simulink model "uz_mpc_3ph"  (R2021a)
settings: Solver=FixedStepDiscrete  StartTime=0.0  StopTime=2000*t_ADC  RelTol=1e-3
values from neighbouring files (symbols this model uses):
  IB = sqrt(2)*IR    [uz_mpc_3ph_init.m]
  id_ref = 0.0    (= 0)    [uz_mpc_3ph_init.m]
  iq_ref = 2.0    (= 2)    [uz_mpc_3ph_init.m]
  lambda_d = 1.0    (= 1)    [uz_mpc_3ph_init.m]
  lambda_q = 1.0    (= 1)    [uz_mpc_3ph_init.m]
  lambda_u = 0.000013    (= 1.3e-05)    [uz_mpc_3ph_init.m]
  Ld_over_LB = Ld/LB    [uz_mpc_3ph_init.m]
  Lq_over_LB = Lq/LB    [uz_mpc_3ph_init.m]
  n_rpm = 250.0    (= 250)    [uz_mpc_3ph_init.m]
  omegaB = nR*2*pi()/60*p    [uz_mpc_3ph_init.m]
  p = 4    [uz_mpc_3ph_init.m]
  psi_pm_over_psiB = psi_pm/psiB    [uz_mpc_3ph_init.m]
  Rs_over_ZB = Rs/ZB    [uz_mpc_3ph_init.m]
  t_ADC = 1/f_ADC    (= 1e-05)    [uz_mpc_3ph_init.m]
  t_clock = 1/f_clock    (= 1e-08)    [uz_mpc_3ph_init.m]
  Ts_times_ZB_over_Ld = Ts*ZB/Ld    [uz_mpc_3ph_init.m]
  Ts_times_ZB_over_Lq = Ts*ZB/Lq    [uz_mpc_3ph_init.m]
  v_dc = 48.0    (= 48)    [uz_mpc_3ph_init.m]
  VB = sqrt(2/3)*VR    [uz_mpc_3ph_init.m]
libraries: nesl_utility x19, simulink x18, fl_lib x15, ee_lib x7, hdlsllib x2, spsAlphaBetaZerotodq0Lib x1
(part 2 of 3)

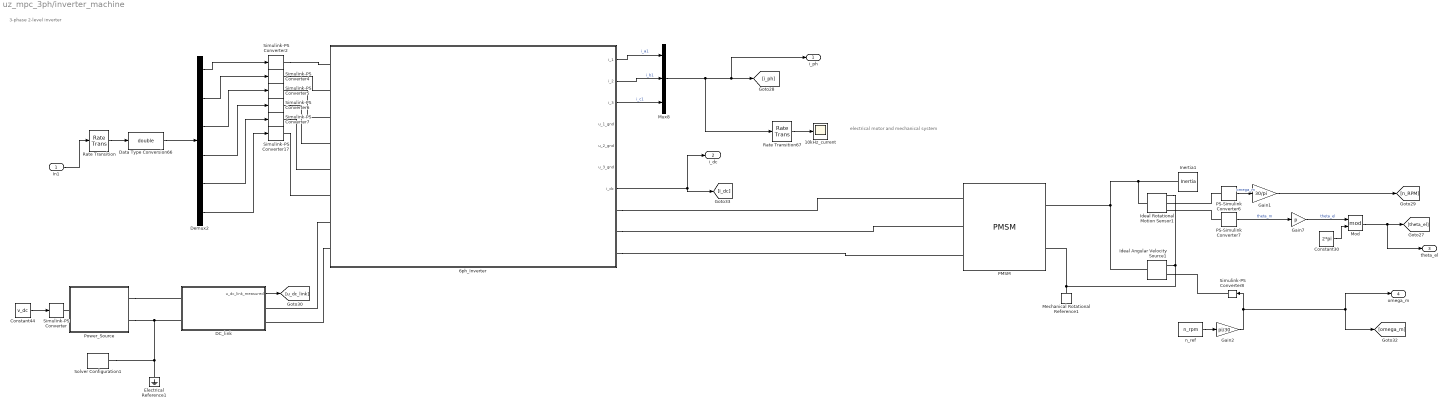
== system uz_mpc_3ph/inverter_machine ==
  note: electrical motor and mechanical system
  note: 3-phase 2-level inverter
  In1 : Inport
  10kHz_current : Scope
  6ph_Inverter : Subsystem
  Constant30 : Constant  Value=2*pi  SampleTime=-1
  Constant44 : Constant  Value=v_dc  SampleTime=-1
  DC_link : Subsystem
  Data Type Conversion66 : DataTypeConversion  OutDataTypeStr=double
  Demux2 : Demux  Outputs=6
  Electrical Reference1 : fl_lib/Electrical/Electrical Elements/Electrical Reference
  Gain1 : Gain  Gain=30/pi
  Gain2 : Gain  Gain=pi/30
  Gain7 : Gain  Gain=p
  Ideal Angular Velocity Source1 : fl_lib/Mechanical/Mechanical Sources/Ideal Angular Velocity Source
  Ideal Rotational Motion Sensor1 : fl_lib/Mechanical/Mechanical Sensors/Ideal Rotational Motion Sensor  wrap_angle=simscape.enum.onoff.off  offset=0 deg
  Inertia1 : fl_lib/Mechanical/Rotational Elements/Inertia  inertia=J kg*m^2  num_ports=foundation.enum.numPorts2.one  w_specify=off  w_priority=High  w=0 rad/s  w_nominal_specify=off  w_nominal_unit=rad/s  w_nominal_value=1  t_specify=off  t_priority=None  t=0 N*m  t_nominal_specify=off  t_nominal_unit=N*m  t_nominal_value=1
  Mechanical Rotational Reference1 : fl_lib/Mechanical/Rotational Elements/Mechanical Rotational Reference
  Mod : Math  Operator=mod  SaturateOnIntegerOverflow=on
  Mux8 : Mux  Inputs=3
  PMSM : ee_lib/Electromechanical/Permanent Magnet/PMSM  winding_type=ee.enum.statorconnection.wye  machine_param=ee.enum.pmsm.parameterization.constant  nPolePairs=p  pmflux_param=ee.enum.pmflux.fluxlinkage  pm_flux_linkage=psi_pm Wb  torque_constant=0.18 N*m/A  back_emf_constant=0.18 V/(rad/s)  stator_param=ee.enum.statorparam.LdLqL0  Ld=Ld H  Lq=Lq H  idVec=[-200, 0, 200] A  iqVec=[-200, 0, 200] A  LdMatrix=0.0002 * ones(3, 3) H  LqMatrix=0.0002 * ones(3, 3) H  PmMatrix=0.1 * ones(3, 3) Wb  ktMatrix=0.18 * ones(3, 3) N*m/A  keMatrix=0.18 * ones(3, 3) V/(rad/s)  L0=0.00016 H  Ls=0.0002 H  Lm=-0.00002 H  Ms=0.00002 H  Rs=Rs Ohm  zero_sequence=ee.enum.park.zerosequence.exclude  J=0.01 kg*m^2  lam=0 N*m/(rad/s)  axes_param=ee.enum.rotorangle.daxis  i_d_specify=off  i_d_priority=None  i_d=0 A  i_d_nominal_specify=off  i_d_nominal_unit=A  i_d_nominal_value=1  i_q_specify=off  i_q_priority=None  i_q=0 A  i_q_nominal_specify=off  i_q_nominal_unit=A  i_q_nominal_value=1  torque_specify=off  torque_priority=None  torque=0 N*m  torque_nominal_specify=off  torque_nominal_unit=N*m  torque_nominal_value=1  angular_velocity_specify=off  angular_velocity_priority=High  angular_velocity=0 rpm  angular_velocity_nominal_specify=off  angular_velocity_nominal_unit=rpm  angular_velocity_nominal_value=1  angular_position_specify=off  angular_position_priority=High  angular_position=0 deg  angular_position_nominal_specify=off  angular_position_nominal_unit=deg  angular_position_nominal_value=1  loss_param=ee.enum.ironloss.none  losses_oc=[0, 0, 0] W  losses_sc=[0, 0, 0] W  f_losses=60 Hz  Isc_losses=95 A  Tmeas=298.15 K  alpha=3.93e-3 1/K  alpha_flux=-0.001 1/K  stator_thermal_mass=100 J/K  rotor_thermal_mass=200 J/K  Rm_percent_rotor=90  Rd_percent_rotor=30  temperatureA_specify=off  temperatureA_priority=High  temperatureA=25 degC  temperatureA_nominal_specify=off  temperatureA_nominal_unit=degC  temperatureA_nominal_value=1  temperatureB_specify=off  temperatureB_priority=High  temperatureB=25 degC  temperatureB_nominal_specify=off  temperatureB_nominal_unit=degC  temperatureB_nominal_value=1  temperatureC_specify=off  temperatureC_priority=High  temperatureC=25 degC  temperatureC_nominal_specify=off  temperatureC_nominal_unit=degC  temperatureC_nominal_value=1  temperatureR_specify=off  temperatureR_priority=High  temperatureR=25 degC  temperatureR_nominal_specify=off  temperatureR_nominal_unit=degC  temperatureR_nominal_value=1
      settings: InternalSimscapePortConfiguration="{\"Bottom\":[],\"Left\":[{\"id\":\"a\",\"label\":\"a\",\"type\":\"foundation.electrical.electrical\"},{\"id\":\"b\",\"label\":\"b\",\"type\":\"foundation.electrical.electrical\"},{\"id\":\"c\",\"label\":\"c\",\"type\":\"foundation.electrical.electrical\"}],\"Right\":[{\"id\":\"R\",\"label\":\"R\",\"type\":\"foundation.mechanical.rotational.rotational\"},{\"id\":\"C\",\"label\":\"C\",\"type\":\"foundation.mechanical.rotational.rotational\"}],\"Top\":[]}"
  PS-Simulink Converter6 : nesl_utility/PS-Simulink Converter  PhysicalDomain=network_engine_domain  SubClassName=ps_output  LeftPortType=input  RightPortType=output  PseudoPeriodic=off  Frequencies=[]  Unit=1  AffineConversion=off
      settings: SourceProductBaseCode=PW,SS
  PS-Simulink Converter7 : nesl_utility/PS-Simulink Converter  PhysicalDomain=network_engine_domain  SubClassName=ps_output  LeftPortType=input  RightPortType=output  PseudoPeriodic=off  Frequencies=[]  Unit=1  AffineConversion=off
      settings: SourceProductBaseCode=PW,SS
  Power_Source : Subsystem
  Rate Transition : RateTransition  OutPortSampleTime=1e-6
  Rate Transition67 : RateTransition  OutPortSampleTime=0.0001
  Simulink-PS Converter{,2,4..8,17} (8 alike) : nesl_utility/Simulink-PS Converter  PhysicalDomain=network_engine_domain  SubClassName=ps_input  LeftPortType=input  RightPortType=output  PseudoPeriodic=off  Frequencies=[]  NoiseDistribution=none  NoiseParameters=[]  Unit=1  AffineConversion=off  FilteringAndDerivatives=provide  SimscapeFilterOrder=1  InputFilterTimeConstant=0.001  UdotUserProvided=0
      Simulink-PS Converter settings: SourceProductBaseCode=PW,SS
      Simulink-PS Converter8 settings: SourceProductBaseCode=PW,SS
  Solver Configuration1 : nesl_utility/Solver Configuration  PhysicalDomain=network_engine_domain  SubClassName=solver  LeftPortType=input  RightPortType=generic  Tones=[]  Harmonics=[]  SimulateNoise=off  Profile=off  UseLocalSampling=off  EnableSwitchedLinearOptims=on  FrequencyDomain=off  UseCCode=off  RelTol=0.001  AbsTol=1e-06  MinStep=1e-09  ToWorkspace=off  RevertToSquareIcSolve=off  NumHomotopyIterations=100  PhasorMode=off  PhasorModeNumHarmonics=1  DoDC=off  ResidualTolerance=1e-09  UseLocalSolver=on  LocalSolverChoice=NE_BACKWARD_EULER_ADVANCER  LocalSolverSampleTime=1e-6  DoFixedCost=on  MaxNonlinIter=3  MaxModeIter=2  ComputeImpulses=off  ImpulseIterations=2  LinearAlgebra=Sparse  EquationFormulation=NE_TIME_EF  DelaysMemoryBudget=1024  AutomaticFiltering=on  FilteringTimeConstant=0.001  PartitionStorageMethod=AS_NEEDED  PartitionMemoryBudget=1024  PartitionMethod=FAST
      settings: SourceProductBaseCode=PW,SS
  n_ref : Constant  Value=n_rpm  SampleTime=-1
  i_ph : Outport
  i_dc : Outport  Port=2
  theta_el : Outport  Port=3
  omega_m : Outport  Port=4
  wires:
  Mux8/1 -> Rate Transition67/1, i_ph/1, [i_ph]
  Gain2/1 -> [omega_m], omega_m/1, Simulink-PS Converter8/1
  Gain7/1 -> Mod/1  "theta_el"
  6ph_Inverter/3(i_3) -> Mux8/3  "i_c1"
  PS-Simulink Converter6/1 -> Gain1/1  "omega_m"
  Gain1/1 -> [n_RPM]
  Demux2/6 -> Simulink-PS Converter17/1
  Demux2/5 -> Simulink-PS Converter7/1
  6ph_Inverter/7(i_dc) -> [i_dc], i_dc/1
  PS-Simulink Converter7/1 -> Gain7/1  "theta_m"
  Data Type Conversion66/1 -> Demux2/1
  Mod/1 -> theta_el/1, [theta_el]
  6ph_Inverter/2(i_2) -> Mux8/2  "i_b1"
  DC_link/1(u_dc_link_measured) -> [u_dc_link]
  In1/1 -> Rate Transition/1
  Demux2/4 -> Simulink-PS Converter6/1
  Constant30/1 -> Mod/2
  6ph_Inverter/1(i_1) -> Mux8/1  "i_a1"
  Constant44/1 -> Simulink-PS Converter/1
  Demux2/1 -> Simulink-PS Converter2/1
  Demux2/2 -> Simulink-PS Converter4/1
  Rate Transition/1 -> Data Type Conversion66/1
  n_ref/1 -> Gain2/1
  Demux2/3 -> Simulink-PS Converter5/1
  Rate Transition67/1 -> 10kHz_current/1
  connections:
  Simulink-PS Converter6/RConn1 -- 6ph_Inverter/LConn4
  PS-Simulink Converter6/LConn1 -- Ideal Rotational Motion Sensor1/RConn2
  Electrical Reference1/LConn1 -- DC_link/LConn2 -- Power_Source/RConn2 -- Solver Configuration1/RConn1
  Ideal Rotational Motion Sensor1/LConn1 -- Ideal Angular Velocity Source1/LConn1 -- PMSM/RConn1 -- Inertia1/LConn1
  Mechanical Rotational Reference1/LConn1 -- PMSM/RConn2 -- Ideal Rotational Motion Sensor1/RConn1 -- Ideal Angular Velocity Source1/RConn2
  6ph_Inverter/RConn3 -- PMSM/LConn3
  6ph_Inverter/LConn8 -- DC_link/RConn2
  Simulink-PS Converter17/RConn1 -- 6ph_Inverter/LConn6
  Simulink-PS Converter7/RConn1 -- 6ph_Inverter/LConn5
  6ph_Inverter/RConn2 -- PMSM/LConn2
  Simulink-PS Converter/RConn1 -- Power_Source/LConn1
  PS-Simulink Converter7/LConn1 -- Ideal Rotational Motion Sensor1/RConn3
  Simulink-PS Converter5/RConn1 -- 6ph_Inverter/LConn3
  Simulink-PS Converter4/RConn1 -- 6ph_Inverter/LConn2
  Simulink-PS Converter8/RConn1 -- Ideal Angular Velocity Source1/RConn1
  Power_Source/RConn1 -- DC_link/LConn1
  6ph_Inverter/LConn7 -- DC_link/RConn1
  6ph_Inverter/RConn1 -- PMSM/LConn1
  Simulink-PS Converter2/RConn1 -- 6ph_Inverter/LConn1

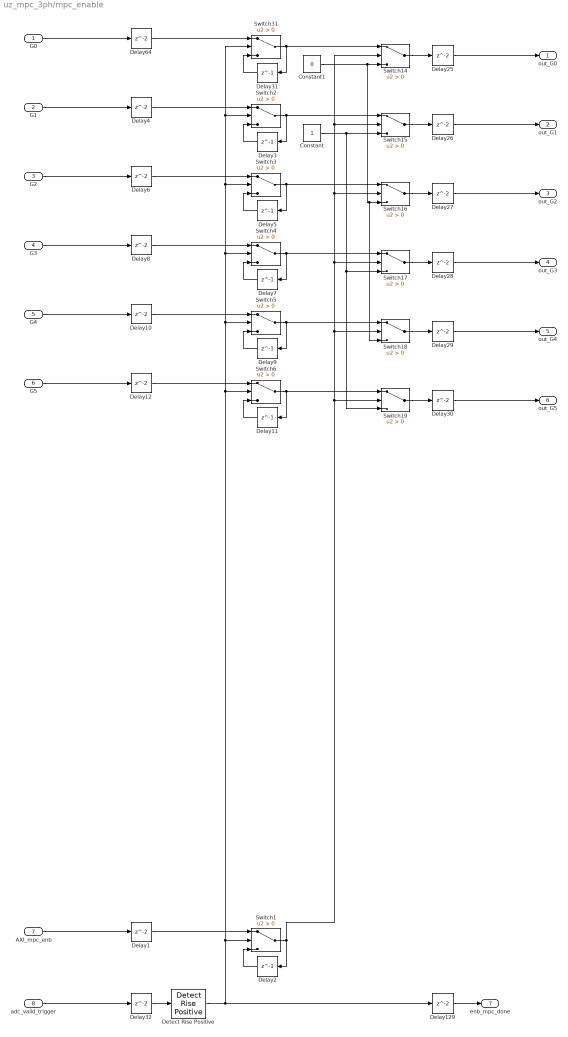
== system uz_mpc_3ph/mpc_enable ==
  G0 : Inport
  G1 : Inport  Port=2
  G2 : Inport  Port=3
  G3 : Inport  Port=4
  G4 : Inport  Port=5
  G5 : Inport  Port=6
  AXI_mpc_enb : Inport  Port=7
  adc_valid_trigger : Inport  Port=8  OutDataTypeStr=boolean
  Constant : Constant  OutDataTypeStr=boolean  SampleTime=-1
  Constant1 : Constant  Value=0  OutDataTypeStr=boolean  SampleTime=-1
  Delay{1,4,6,8,10,12,25..30,32,64,129} (15 alike) : Delay
  Delay{2..3,5,7,9,11,31} (7 alike) : Delay  DelayLength=1
  Detect Rise Positive : simulink/Logic and Bit Operations/Detect Rise Positive  vinit=0  OutDataTypeStr=boolean
  Switch{1..6,14..19,31} (13 alike) : Switch  Criteria=u2 > Threshold
  out_G0 : Outport
  out_G1 : Outport  Port=2
  out_G2 : Outport  Port=3
  out_G3 : Outport  Port=4
  out_G4 : Outport  Port=5
  out_G5 : Outport  Port=6
  enb_mpc_done : Outport  Port=7  OutDataTypeStr=boolean  LockScale=on
  wires:
  adc_valid_trigger/1 -> Delay32/1
  G0/1 -> Delay64/1
  Delay129/1 -> enb_mpc_done/1
  Delay64/1 -> Switch31/1
  Delay32/1 -> Detect Rise Positive/1
  Switch31/1 -> Switch14/1, Delay31/1
  Delay31/1 -> Switch31/3
  AXI_mpc_enb/1 -> Delay1/1
  Delay1/1 -> Switch1/1
  Delay2/1 -> Switch1/3
  Delay3/1 -> Switch2/3
  Switch2/1 -> Switch15/1, Delay3/1
  Delay4/1 -> Switch2/1
  G1/1 -> Delay4/1
  Detect Rise Positive/1 -> Delay129/1, Switch31/2, Switch2/2, Switch3/2, Switch4/2, Switch5/2, Switch6/2, Switch1/2
  Delay5/1 -> Switch3/3
  Switch3/1 -> Switch16/1, Delay5/1
  Delay6/1 -> Switch3/1
  G2/1 -> Delay6/1
  Delay7/1 -> Switch4/3
  Switch4/1 -> Switch17/1, Delay7/1
  Delay8/1 -> Switch4/1
  G3/1 -> Delay8/1
  Delay9/1 -> Switch5/3
  Switch5/1 -> Switch18/1, Delay9/1
  Delay10/1 -> Switch5/1
  G4/1 -> Delay10/1
  Delay11/1 -> Switch6/3
  Switch6/1 -> Switch19/1, Delay11/1
  Delay12/1 -> Switch6/1
  G5/1 -> Delay12/1
  Switch14/1 -> Delay25/1
  Delay25/1 -> out_G0/1
  Constant1/1 -> Switch18/3, Switch16/3, Switch14/3
  Switch15/1 -> Delay26/1
  Delay26/1 -> out_G1/1
  Switch1/1 -> Switch19/2, Switch18/2, Switch17/2, Switch16/2, Switch15/2, Switch14/2, Delay2/1
  Switch16/1 -> Delay27/1
  Delay28/1 -> out_G3/1
  Switch17/1 -> Delay28/1
  Delay27/1 -> out_G2/1
  Delay29/1 -> out_G4/1
  Switch19/1 -> Delay30/1
  Switch18/1 -> Delay29/1
  Delay30/1 -> out_G5/1
  Constant/1 -> Switch19/3, Switch17/3, Switch15/3

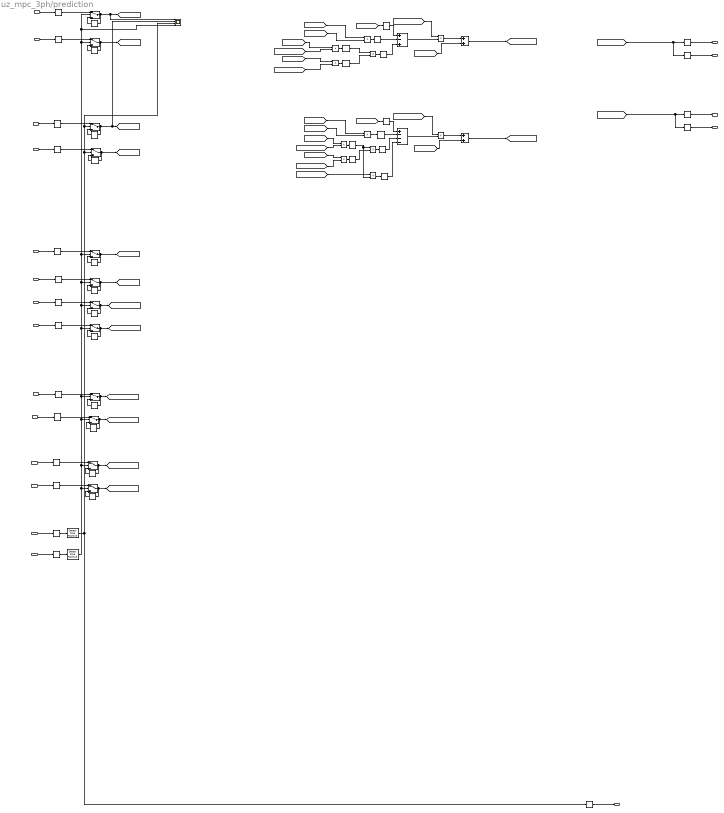
== system uz_mpc_3ph/prediction ==
  note: voltages are triggered every iteration
  note: iq_delay_pu = Ts_times_ZB_over_Lq *(vq_pu - Rs_over_ZB * iq_k_pu - omega_m_pu * polepairs * Ld_over_LB * id_k_pu - omega_m_pu * polepairs * psi_pm_over_psiB) + iq_k_pu
  note: id_delay_pu = Ts_times_ZB_over_Ld *(vd_pu - Rs_over_ZB * id_k_pu + iq_k_pu * Lq_over_LB * omega_m_pu * polepairs) + id_k_pu
  id_delay_pu : Inport  OutDataTypeStr=fixdt_type_dq_currents
  iq_delay_pu : Inport  Port=2  OutDataTypeStr=fixdt_type_dq_currents
  vd_pu : Inport  Port=3  OutDataTypeStr=fixdt_type_dqxy_voltages
  vq_pu : Inport  Port=4  OutDataTypeStr=fixdt_type_dqxy_voltages
  omega_m_pu : Inport  Port=5  OutDataTypeStr=fixdt_type_speed
  Rs_over_ZB_AXI : Inport  Port=6  OutDataTypeStr=fixdt_type_constants
  Ts_times_ZB_over_Ld_AXI : Inport  Port=7  OutDataTypeStr=fixdt_type_constants
  Ts_times_ZB_over_Lq_AXI : Inport  Port=8  OutDataTypeStr=fixdt_type_constants
  Ld_over_LB_AXI : Inport  Port=9  OutDataTypeStr=fixdt_type_constants
  Lq_over_LB_AXI : Inport  Port=10  OutDataTypeStr=fixdt_type_constants
  psi_pm_over_psiB_AXI : Inport  Port=11  OutDataTypeStr=fixdt_type_constants
  polepairs_AXI : Inport  Port=12  OutDataTypeStr=fixdt_type_polepairs
  trigger_prediction : Inport  Port=13
  trigger_delay_comp_done : Inport  Port=14
  Add : Sum  Inputs=+-+  AccumDataTypeStr=fixdt(1,27,16)
  Add1 : Sum  AccumDataTypeStr=fixdt(1,27,24)
  Add2 : Sum  Inputs=+---  AccumDataTypeStr=fixdt(1,27,16)
  Add3 : Sum  AccumDataTypeStr=fixdt(1,27,24)
  Delay{,2,4,11..12,14..15,25,27,29,35,37,39,43,50,59..60,62..63} (19 alike) : Delay
  Delay{1,3,5,10,13,18..22,26,28,30,36,38,40,44..48,57..58} (23 alike) : Delay  DelayLength=1
  Detect Rise Positive : simulink/Logic and Bit Operations/Detect Rise Positive  vinit=0  OutDataTypeStr=boolean
  Detect Rise Positive1 : simulink/Logic and Bit Operations/Detect Rise Positive  vinit=0  OutDataTypeStr=boolean
  Product{,1..2,4..7,9..10} (9 alike) : Product  OutDataTypeStr=fixdt(1,18,15)
  Product3 : Product  OutDataTypeStr=fixdt(1,27,16)
  Product8 : Product  OutDataTypeStr=fixdt(1,27,16)
  Scope : Scope  NumInputPorts=4
  Switch : Switch  Criteria=u2 > Threshold  OutDataTypeStr=fixdt_type_dq_currents
  Switch1 : Switch  Criteria=u2 > Threshold  OutDataTypeStr=fixdt_type_dq_currents
  Switch{12..14,17..19} (6 alike) : Switch  Criteria=u2 > Threshold  OutDataTypeStr=fixdt_type_constants
  Switch21 : Switch  Criteria=u2 > Threshold  OutDataTypeStr=fixdt_type_polepairs
  Switch28 : Switch  Criteria=u2 > Threshold  OutDataTypeStr=fixdt_type_dqxy_voltages
  Switch29 : Switch  Criteria=u2 > Threshold  OutDataTypeStr=fixdt_type_dqxy_voltages
  Switch5 : Switch  Criteria=u2 > Threshold  OutDataTypeStr=fixdt_type_speed
  id_pred_pu : Outport
  iq_pred_pu : Outport  Port=2
  id_pred_pu_AXI : Outport  Port=3
  iq_pred_pu_AXI : Outport  Port=4
  prediction_done : Outport  Port=5
  wires:
  Switch12/1 -> [Rs_over_ZB_AXI], Delay26/1
  Add3/1 -> [iq_delay_pu]
  Add1/1 -> [id_delay_pu]
  Delay5/1 -> Switch1/3
  Delay25/1 -> Switch12/1
  Delay59/1 -> Switch28/1
  vd_pu/1 -> Delay59/1
  Ld_over_LB_AXI/1 -> Delay35/1
  Delay2/1 -> Switch/1
  Delay38/1 -> Switch18/3
  Switch17/1 -> Delay36/1, [Ld_over_LB_AXI]
  Switch13/1 -> [Ts_times_ZB_over_Ld_AXI], Delay28/1
  Delay/1 -> Detect Rise Positive/1
  Delay44/1 -> Switch21/3
  Delay29/1 -> Switch14/1
  Switch29/1 -> [vq_pu], Delay58/1
  polepairs_AXI/1 -> Delay43/1
  Delay43/1 -> Switch21/1
  Switch14/1 -> [Ts_times_ZB_over_Lq_AXI], Delay30/1
  Delay28/1 -> Switch13/3
  psi_pm_over_psiB_AXI/1 -> Delay39/1
  Delay58/1 -> Switch29/3
  id_delay_pu/1 -> Delay2/1
  Switch21/1 -> [polepairs_AXI], Delay44/1
  Switch/1 -> Scope/1, [id_pu], Delay3/1
  Delay35/1 -> Switch17/1
  Switch28/1 -> Scope/2, [vd_pu], Delay57/1
  Delay37/1 -> Switch18/1
  Delay4/1 -> Switch1/1
  Delay12/1 -> Switch5/1
  omega_m_pu/1 -> Delay12/1
  Delay27/1 -> Switch13/1
  vq_pu/1 -> Delay60/1
  Switch5/1 -> [omega_m_pu], Delay13/1
  Lq_over_LB_AXI/1 -> Delay37/1
  iq_delay_pu/1 -> Delay4/1
  Delay60/1 -> Switch29/1
  Ts_times_ZB_over_Lq_AXI/1 -> Delay29/1
  Delay3/1 -> Switch/3
  Switch18/1 -> Delay38/1, [Lq_over_LB_AXI]
  Delay26/1 -> Switch12/3
  Switch19/1 -> [psi_pm_over_psiB_AXI], Delay40/1
  Switch1/1 -> [iq_pu], Delay5/1
  Ts_times_ZB_over_Ld_AXI/1 -> Delay27/1
  Delay57/1 -> Switch28/3
  Rs_over_ZB_AXI/1 -> Delay25/1
  Delay39/1 -> Switch19/1
  trigger_delay_comp_done/1 -> Delay/1
  Delay40/1 -> Switch19/3
  Delay13/1 -> Switch5/3
  Delay36/1 -> Switch17/3
  Delay30/1 -> Switch14/3
  Delay11/1 -> prediction_done/1
  [iq_delay_pu] -> Delay15/1, Delay63/1
  [id_delay_pu] -> Delay14/1, Delay62/1
  Delay63/1 -> iq_pred_pu_AXI/1
  Delay62/1 -> id_pred_pu_AXI/1
  Delay15/1 -> iq_pred_pu/1
  Delay14/1 -> id_pred_pu/1
  Add/1 -> Product/2
  [Ts_times_ZB_over_Ld_AXI] -> Product/1  "Ts_times_ZB_over_Ld"
  Product/1 -> Add1/1
  [id_pu] -> Add1/2  "id_k_pu"
  [Rs_over_ZB_AXI] -> Product1/1  "Rs_over_ZB"
  [id_pu] -> Product1/2  "id_k_pu"
  [iq_pu] -> Product3/1  "iq_k_pu"
  [Lq_over_LB_AXI] -> Product3/2  "Lq_over_LB"
  [omega_m_pu] -> Product4/1  "omega_m_pu"
  [polepairs_AXI] -> Product4/2  "polepairs"
  [Ts_times_ZB_over_Lq_AXI] -> Product5/1  "Ts_times_ZB_over_Lq"
  [iq_pu] -> Product6/2  "iq_k_pu"
  [Rs_over_ZB_AXI] -> Product6/1  "Rs_over_ZB"
  Add2/1 -> Product5/2
  [omega_m_pu] -> Product9/1  "omega_m_pu"
  [iq_pu] -> Add3/2  "iq_k_pu"
  [id_pu] -> Product8/1  "id_k_pu"
  [Ld_over_LB_AXI] -> Product8/2  "Ld_over_LB"
  [polepairs_AXI] -> Product9/2  "polepairs"
  Product5/1 -> Add3/1
  [psi_pm_over_psiB_AXI] -> Product10/1
  Product2/1 -> Delay1/1
  Product1/1 -> Delay10/1
  Delay10/1 -> Add/2
  Delay1/1 -> Add/3
  [vd_pu] -> Delay18/1  "vd_pu"
  Delay18/1 -> Add/1
  [vq_pu] -> Delay19/1  "vq_pu"
  Product7/1 -> Delay21/1
  Product10/1 -> Delay22/1
  Delay22/1 -> Add2/4
  Delay21/1 -> Add2/3
  Delay20/1 -> Add2/2
  Delay19/1 -> Add2/1
  Product6/1 -> Delay20/1
  Product4/1 -> Delay45/1
  Product3/1 -> Delay46/1
  Delay46/1 -> Product2/2
  Delay45/1 -> Product2/1
  Product9/1 -> Delay47/1
  Delay47/1 -> Product10/2, Product7/1
  Product8/1 -> Delay48/1
  Delay48/1 -> Product7/2
  Detect Rise Positive1/1 -> Delay11/1, Switch29/2, Scope/3, Switch28/2  "delay_comp done"
  trigger_prediction/1 -> Delay50/1
  Delay50/1 -> Detect Rise Positive1/1
  Detect Rise Positive/1 -> Switch21/2, Switch19/2, Switch18/2, Switch17/2, Switch14/2, Switch13/2, Switch12/2, Switch5/2, Switch1/2, Scope/4, Switch/2

== system uz_mpc_3ph/pu_omega_m ==
  in1 : Inport  OutDataTypeStr=fixdt(1,24,11)
  AXI_pu_conv_in : Inport  Port=2  OutDataTypeStr=fixdt(0,18,18)
  adc_valid_trigger : Inport  Port=3  OutDataTypeStr=boolean
  Delay{32,64,127..129} (5 alike) : Delay
  Delay31 : Delay  DelayLength=1
  Detect Rise Positive : simulink/Logic and Bit Operations/Detect Rise Positive  vinit=0  OutDataTypeStr=boolean
  Product23 : Product  OutDataTypeStr=fixdt(1,24,11)
  Switch31 : Switch  Criteria=u2 > Threshold
  out1 : Outport
  pu_conv_done : Outport  Port=2  OutDataTypeStr=boolean  LockScale=on
  out1_AXI : Outport  Port=3
  wires:
  adc_valid_trigger/1 -> Delay32/1
  in1/1 -> Delay64/1
  Delay129/1 -> pu_conv_done/1
  AXI_pu_conv_in/1 -> Product23/1
  Delay64/1 -> Switch31/1
  Delay128/1 -> out1_AXI/1
  Delay32/1 -> Detect Rise Positive/1
  Switch31/1 -> Product23/2, Delay31/1
  Delay31/1 -> Switch31/3
  Detect Rise Positive/1 -> Delay129/1, Switch31/2
  Product23/1 -> Delay127/1, Delay128/1
  Delay127/1 -> out1/1

== system uz_mpc_3ph/pu_omega_m1 ==
  in1 : Inport  OutDataTypeStr=fixdt(1,24,11)
  AXI_pu_conv_in : Inport  Port=2  OutDataTypeStr=fixdt(0,18,18)
  adc_valid_trigger : Inport  Port=3  OutDataTypeStr=boolean
  Delay{32,64,127..129} (5 alike) : Delay
  Delay31 : Delay  DelayLength=1
  Detect Rise Positive : simulink/Logic and Bit Operations/Detect Rise Positive  vinit=0  OutDataTypeStr=boolean
  Product23 : Product  OutDataTypeStr=fixdt(1,24,11)
  Switch31 : Switch  Criteria=u2 > Threshold
  out1 : Outport
  pu_conv_done : Outport  Port=2  OutDataTypeStr=boolean  LockScale=on
  out1_AXI : Outport  Port=3
  wires:
  adc_valid_trigger/1 -> Delay32/1
  in1/1 -> Delay64/1
  Delay129/1 -> pu_conv_done/1
  AXI_pu_conv_in/1 -> Product23/1
  Delay64/1 -> Switch31/1
  Delay128/1 -> out1_AXI/1
  Delay32/1 -> Detect Rise Positive/1
  Switch31/1 -> Product23/2, Delay31/1
  Delay31/1 -> Switch31/3
  Detect Rise Positive/1 -> Delay129/1, Switch31/2
  Product23/1 -> Delay127/1, Delay128/1
  Delay127/1 -> out1/1

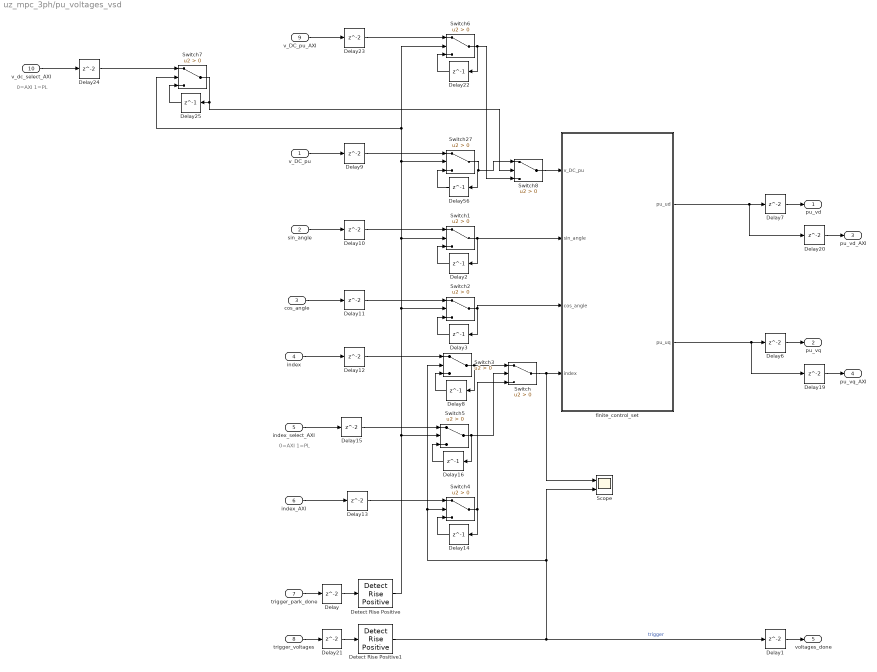
== system uz_mpc_3ph/pu_voltages_vsd ==
  note: 0=AXI 1=PL
  note: 0=AXI 1=PL
  v_DC_pu : Inport  OutDataTypeStr=fixdt_type_constants
  sin_angle : Inport  Port=2  OutDataTypeStr=fixdt_type_sin_cos
  cos_angle : Inport  Port=3  OutDataTypeStr=fixdt_type_sin_cos
  index : Inport  Port=4
  index_select_AXI : Inport  Port=5
  index_AXI : Inport  Port=6
  trigger_park_done : Inport  Port=7
  trigger_voltages : Inport  Port=8
  v_DC_pu_AXI : Inport  Port=9  OutDataTypeStr=fixdt_type_constants
  v_dc_select_AXI : Inport  Port=10
  Delay{,1,6..7,9..11,19..21,23} (11 alike) : Delay
  Delay{12..13,15,24} (4 alike) : Delay  InitialCondition=1
  Delay{8,14,16,25} (4 alike) : Delay  DelayLength=1  InitialCondition=1
  Delay{2..3,22,56} (4 alike) : Delay  DelayLength=1
  Detect Rise Positive : simulink/Logic and Bit Operations/Detect Rise Positive  vinit=0  OutDataTypeStr=boolean
  Detect Rise Positive1 : simulink/Logic and Bit Operations/Detect Rise Positive  vinit=0  OutDataTypeStr=boolean
  Scope : Scope  NumInputPorts=2
  Switch : Switch  Criteria=u2 > Threshold
  Switch1 : Switch  Criteria=u2 > Threshold  OutDataTypeStr=fixdt_type_sin_cos
  Switch2 : Switch  Criteria=u2 > Threshold  OutDataTypeStr=fixdt_type_sin_cos
  Switch27 : Switch  Criteria=u2 > Threshold  OutDataTypeStr=fixdt_type_constants
  Switch{3..5,7} (4 alike) : Switch  Criteria=u2 > Threshold  OutDataTypeStr=fixdt_type_polepairs
  Switch6 : Switch  Criteria=u2 > Threshold  OutDataTypeStr=fixdt_type_constants
  Switch8 : Switch  Criteria=u2 > Threshold
  finite_control_set : MATLAB Function  TreatAsAtomicUnit=on
  pu_vd : Outport
  pu_vq : Outport  Port=2
  pu_vd_AXI : Outport  Port=3
  pu_vq_AXI : Outport  Port=4
  voltages_done : Outport  Port=5
  wires:
  finite_control_set/1(pu_ud) -> Delay7/1, Delay20/1
  finite_control_set/2(pu_uq) -> Delay6/1, Delay19/1
  trigger_park_done/1 -> Delay/1
  Delay/1 -> Detect Rise Positive/1
  Delay56/1 -> Switch27/3
  v_DC_pu/1 -> Delay9/1
  Switch27/1 -> Switch8/1, Delay56/1
  sin_angle/1 -> Delay10/1
  Delay2/1 -> Switch1/3
  Switch1/1 -> finite_control_set/2(sin_angle), Delay2/1
  cos_angle/1 -> Delay11/1
  Delay3/1 -> Switch2/3
  Switch2/1 -> finite_control_set/3(cos_angle), Delay3/1
  Delay6/1 -> pu_vq/1
  Delay7/1 -> pu_vd/1
  Switch3/1 -> Delay8/1, Switch/1
  index/1 -> Delay12/1
  Delay8/1 -> Switch3/3
  Delay9/1 -> Switch27/1
  Delay10/1 -> Switch1/1
  Delay11/1 -> Switch2/1
  Delay12/1 -> Switch3/1
  Delay14/1 -> Switch4/3
  index_AXI/1 -> Delay13/1
  Switch4/1 -> Switch/3, Delay14/1
  Delay13/1 -> Switch4/1
  Delay16/1 -> Switch5/3
  index_select_AXI/1 -> Delay15/1
  Switch5/1 -> Switch/2, Delay16/1
  Delay15/1 -> Switch5/1
  Delay19/1 -> pu_vq_AXI/1
  Delay20/1 -> pu_vd_AXI/1
  Detect Rise Positive1/1 -> Delay1/1, Scope/2, Switch3/2, Switch4/2  "trigger"
  Delay1/1 -> voltages_done/1
  trigger_voltages/1 -> Delay21/1
  Delay21/1 -> Detect Rise Positive1/1
  Switch/1 -> Scope/1, finite_control_set/4(index)
  Switch6/1 -> Switch8/3, Delay22/1
  Delay22/1 -> Switch6/3
  v_DC_pu_AXI/1 -> Delay23/1
  Delay23/1 -> Switch6/1
  v_dc_select_AXI/1 -> Delay24/1
  Delay25/1 -> Switch7/3
  Switch7/1 -> Switch8/2, Delay25/1
  Delay24/1 -> Switch7/1
  Detect Rise Positive/1 -> Switch5/2, Switch2/2, Switch7/2, Switch6/2, Switch27/2, Switch1/2
  Switch8/1 -> finite_control_set/1(v_DC_pu)

== system uz_mpc_3ph/uz_clarke ==
  a1 : Inport
  b1 : Inport  Port=2
  c1 : Inport  Port=3
  pu_conv_valid : Inport  Port=4
  Delay : Delay  DelayLength=1
  Delay1 : Delay  DelayLength=1
  Delay{6..9,13..15,20} (8 alike) : Delay
  Delay2 : Delay  DelayLength=1
  Detect Rise Positive : simulink/Logic and Bit Operations/Detect Rise Positive  vinit=0  OutDataTypeStr=boolean
  Switch : Switch  Criteria=u2 > Threshold  OutDataTypeStr=fixdt_type_vsd
  Switch1 : Switch  Criteria=u2 > Threshold  OutDataTypeStr=fixdt_type_vsd
  Switch2 : Switch  Criteria=u2 > Threshold  OutDataTypeStr=fixdt_type_vsd
  Terminator : Terminator
  clarke : MATLAB Function  TreatAsAtomicUnit=on
  alpha : Outport  OutDataTypeStr=fixdt(1,18,11)  VectorParamsAs1DForOutWhenUnconnected=off
  beta : Outport  Port=2  OutDataTypeStr=fixdt(1,18,11)  VectorParamsAs1DForOutWhenUnconnected=off
  clarke_done : Outport  Port=3  VectorParamsAs1DForOutWhenUnconnected=off
  alpha_AXI : Outport  Port=4  OutDataTypeStr=fixdt(1,18,11)  VectorParamsAs1DForOutWhenUnconnected=off
  beta_AXI : Outport  Port=5  OutDataTypeStr=fixdt(1,18,11)  VectorParamsAs1DForOutWhenUnconnected=off
  wires:
  clarke/1(alpha) -> Delay20/1, Delay14/1
  pu_conv_valid/1 -> Delay6/1
  Detect Rise Positive/1 -> Switch2/2, Switch1/2, Switch/2, Delay13/1
  Delay/1 -> Switch/3
  Switch/1 -> clarke/1(a1), Delay/1
  Delay1/1 -> Switch1/3
  Switch1/1 -> clarke/2(b1), Delay1/1
  Delay2/1 -> Switch2/3
  Switch2/1 -> Delay2/1, clarke/3(c1)
  a1/1 -> Delay7/1
  b1/1 -> Delay8/1
  c1/1 -> Delay9/1
  Delay6/1 -> Detect Rise Positive/1
  Delay7/1 -> Switch/1
  Delay8/1 -> Switch1/1
  Delay9/1 -> Switch2/1
  Delay13/1 -> clarke_done/1
  Delay14/1 -> alpha/1
  Delay15/1 -> beta/1
  Delay20/1 -> alpha_AXI/1
  clarke/2(beta) -> beta_AXI/1, Delay15/1
  clarke/3(zero) -> Terminator/1

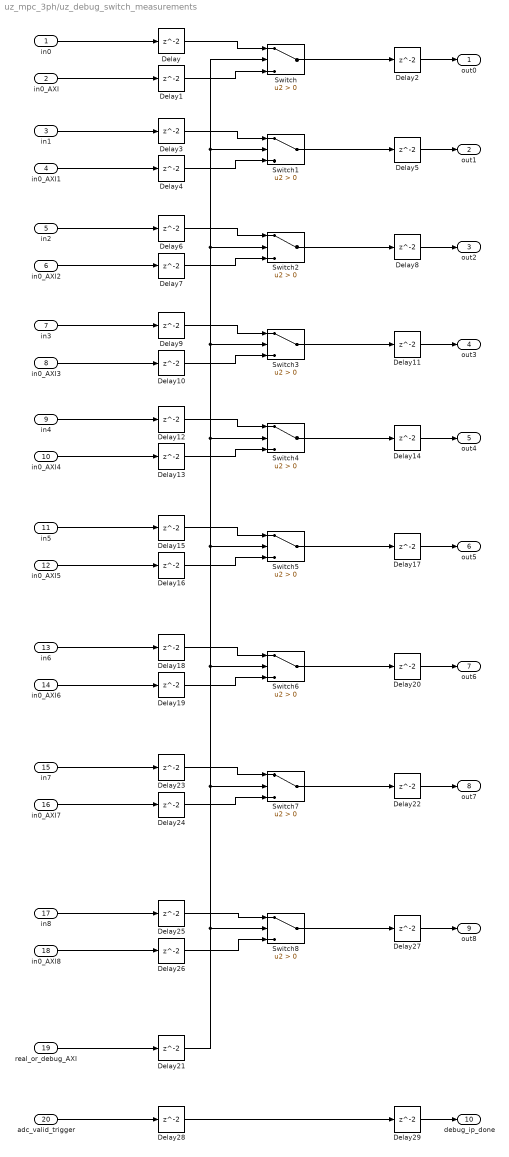
== system uz_mpc_3ph/uz_debug_switch_measurements ==
  in0 : Inport
  in0_AXI : Inport  Port=2
  in1 : Inport  Port=3
  in0_AXI1 : Inport  Port=4
  in2 : Inport  Port=5
  in0_AXI2 : Inport  Port=6
  in3 : Inport  Port=7
  in0_AXI3 : Inport  Port=8
  in4 : Inport  Port=9
  in0_AXI4 : Inport  Port=10
  in5 : Inport  Port=11
  in0_AXI5 : Inport  Port=12
  in6 : Inport  Port=13
  in0_AXI6 : Inport  Port=14
  in7 : Inport  Port=15
  in0_AXI7 : Inport  Port=16
  in8 : Inport  Port=17
  in0_AXI8 : Inport  Port=18
  real_or_debug_AXI : Inport  Port=19
  adc_valid_trigger : Inport  Port=20
  Delay{,1..29} (30 alike) : Delay
  Switch{,1..8} (9 alike) : Switch  Criteria=u2 > Threshold
  out0 : Outport  VectorParamsAs1DForOutWhenUnconnected=off
  out1 : Outport  Port=2  VectorParamsAs1DForOutWhenUnconnected=off
  out2 : Outport  Port=3  VectorParamsAs1DForOutWhenUnconnected=off
  out3 : Outport  Port=4  VectorParamsAs1DForOutWhenUnconnected=off
  out4 : Outport  Port=5  VectorParamsAs1DForOutWhenUnconnected=off
  out5 : Outport  Port=6  VectorParamsAs1DForOutWhenUnconnected=off
  out6 : Outport  Port=7  VectorParamsAs1DForOutWhenUnconnected=off
  out7 : Outport  Port=8  VectorParamsAs1DForOutWhenUnconnected=off
  out8 : Outport  Port=9  VectorParamsAs1DForOutWhenUnconnected=off
  debug_ip_done : Outport  Port=10  VectorParamsAs1DForOutWhenUnconnected=off
  wires:
  in0/1 -> Delay/1
  in0_AXI/1 -> Delay1/1
  Delay/1 -> Switch/1
  Delay1/1 -> Switch/3
  Switch/1 -> Delay2/1
  Delay2/1 -> out0/1
  in0_AXI1/1 -> Delay4/1
  Delay5/1 -> out1/1
  in1/1 -> Delay3/1
  Delay4/1 -> Switch1/3
  Delay3/1 -> Switch1/1
  Switch1/1 -> Delay5/1
  in0_AXI2/1 -> Delay7/1
  Delay8/1 -> out2/1
  in2/1 -> Delay6/1
  Delay7/1 -> Switch2/3
  Delay6/1 -> Switch2/1
  Switch2/1 -> Delay8/1
  in0_AXI3/1 -> Delay10/1
  Delay11/1 -> out3/1
  in3/1 -> Delay9/1
  Delay10/1 -> Switch3/3
  Delay9/1 -> Switch3/1
  Switch3/1 -> Delay11/1
  in0_AXI4/1 -> Delay13/1
  Delay14/1 -> out4/1
  in4/1 -> Delay12/1
  Delay13/1 -> Switch4/3
  Delay12/1 -> Switch4/1
  Switch4/1 -> Delay14/1
  in0_AXI5/1 -> Delay16/1
  Delay17/1 -> out5/1
  in5/1 -> Delay15/1
  Delay16/1 -> Switch5/3
  Delay15/1 -> Switch5/1
  Switch5/1 -> Delay17/1
  in0_AXI6/1 -> Delay19/1
  Delay20/1 -> out6/1
  in6/1 -> Delay18/1
  Delay19/1 -> Switch6/3
  Delay18/1 -> Switch6/1
  Switch6/1 -> Delay20/1
  real_or_debug_AXI/1 -> Delay21/1
  Delay22/1 -> out7/1
  Delay23/1 -> Switch7/1
  Delay24/1 -> Switch7/3
  Switch7/1 -> Delay22/1
  in0_AXI7/1 -> Delay24/1
  in7/1 -> Delay23/1
  in0_AXI8/1 -> Delay26/1
  in8/1 -> Delay25/1
  Delay27/1 -> out8/1
  Switch8/1 -> Delay27/1
  Delay25/1 -> Switch8/1
  Delay26/1 -> Switch8/3
  Delay21/1 -> Switch/2, Switch1/2, Switch2/2, Switch3/2, Switch4/2, Switch5/2, Switch6/2, Switch7/2, Switch8/2
  Delay28/1 -> Delay29/1
  Delay29/1 -> debug_ip_done/1
  adc_valid_trigger/1 -> Delay28/1

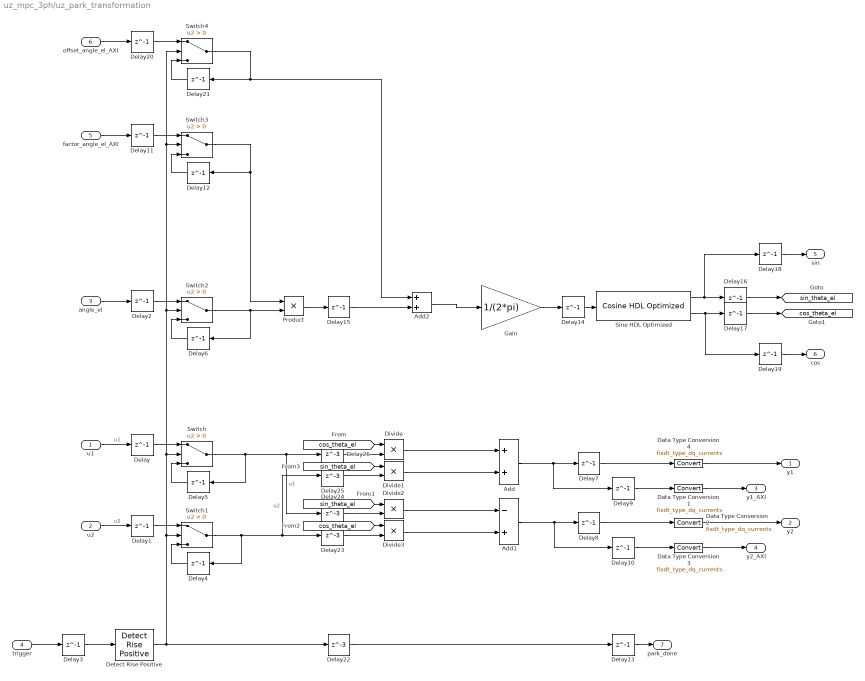
== system uz_mpc_3ph/uz_park_transformation ==
  u1 : Inport
  u2 : Inport  Port=2
  angle_el : Inport  Port=3
  trigger : Inport  Port=4
  factor_angle_el_AXI : Inport  Port=5
  offset_angle_el_AXI : Inport  Port=6
  Add : Sum  OutDataTypeStr=fixdt(1,27,16)
  Add1 : Sum  Inputs=-+  OutDataTypeStr=fixdt(1,27,16)
  Add2 : Sum  AccumDataTypeStr=fixdt(1,27,20)
  Data Type Conversion{1..4} (4 alike) : DataTypeConversion  OutDataTypeStr=fixdt_type_dq_currents
  Delay{,1..21} (22 alike) : Delay  DelayLength=1
  Delay{22..26} (5 alike) : Delay  DelayLength=3
  Detect Rise Positive : simulink/Logic and Bit Operations/Detect Rise Positive  vinit=0  OutDataTypeStr=boolean
  Divide{,1..3} (4 alike) : Product  Inputs=**  OutDataTypeStr=fixdt(1,27,16)
  Gain : Gain  Gain=1/(2*pi)  OutDataTypeStr=fixdt(1,27,20)
  Product : Product  OutDataTypeStr=fixdt(1,27,20)
  Sine HDL Optimized : hdlsllib/Lookup Tables/Cosine HDL Optimized  OutputFormula=sin(2*pi*u) and cos(2*pi*u)  NumDataPoints=256  TableDataTypeStr=fixdt(0,26,20)  SimulateLUTROMDelay=off
      settings: SourceProductBaseCode=SL
  Switch{,1..4} (5 alike) : Switch  Criteria=u2 > Threshold
  y1 : Outport  VectorParamsAs1DForOutWhenUnconnected=off
  y2 : Outport  Port=2  VectorParamsAs1DForOutWhenUnconnected=off
  y1_AXI : Outport  Port=3  VectorParamsAs1DForOutWhenUnconnected=off
  y2_AXI : Outport  Port=4  VectorParamsAs1DForOutWhenUnconnected=off
  sin : Outport  Port=5  VectorParamsAs1DForOutWhenUnconnected=off
  cos : Outport  Port=6  VectorParamsAs1DForOutWhenUnconnected=off
  park_done : Outport  Port=7  VectorParamsAs1DForOutWhenUnconnected=off
  tag scope: cos_theta_el=global, sin_theta_el=global
  wires:
  Switch1/1 -> Delay4/1, Delay25/1, Delay23/1  "u2"
  Divide2/1 -> Add1/1
  Divide3/1 -> Add1/2
  [cos_theta_el] -> Divide3/1
  Switch/1 -> Delay24/1, Delay26/1, Delay5/1  "u1"
  [sin_theta_el] -> Divide2/1
  Divide1/1 -> Add/2
  [cos_theta_el] -> Divide/1
  [sin_theta_el] -> Divide1/1
  Add/1 -> Delay9/1, Delay7/1
  Add1/1 -> Delay10/1, Delay8/1
  Divide/1 -> Add/1
  angle_el/1 -> Delay2/1
  Sine HDL Optimized/2 -> Delay19/1, Delay17/1
  Sine HDL Optimized/1 -> Delay18/1, Delay16/1
  Gain/1 -> Delay14/1
  u1/1 -> Delay/1  "u1"
  u2/1 -> Delay1/1  "u2"
  Delay/1 -> Switch/1
  Delay1/1 -> Switch1/1
  Delay2/1 -> Switch2/1
  trigger/1 -> Delay3/1
  Delay4/1 -> Switch1/3
  Delay5/1 -> Switch/3
  Delay6/1 -> Switch2/3
  Delay7/1 -> Data Type Conversion4/1
  Switch2/1 -> Product/2, Delay6/1
  Switch3/1 -> Product/1, Delay12/1
  factor_angle_el_AXI/1 -> Delay11/1
  Delay12/1 -> Switch3/3
  Delay11/1 -> Switch3/1
  Product/1 -> Delay15/1
  Delay3/1 -> Detect Rise Positive/1
  Delay13/1 -> park_done/1
  Delay14/1 -> Sine HDL Optimized/1
  Delay16/1 -> [sin_theta_el]
  Delay17/1 -> [cos_theta_el]
  Delay18/1 -> sin/1
  Delay19/1 -> cos/1
  Add2/1 -> Gain/1
  Delay20/1 -> Switch4/1
  Switch4/1 -> Add2/1, Delay21/1
  Detect Rise Positive/1 -> Delay22/1, Switch1/2, Switch/2, Switch4/2, Switch3/2, Switch2/2
  Delay21/1 -> Switch4/3
  offset_angle_el_AXI/1 -> Delay20/1
  Delay15/1 -> Add2/2
  Delay22/1 -> Delay13/1
  Delay23/1 -> Divide3/2
  Delay24/1 -> Divide2/2
  Delay25/1 -> Divide1/2
  Delay26/1 -> Divide/2
  Data Type Conversion4/1 -> y1/1
  Delay9/1 -> Data Type Conversion1/1
  Delay8/1 -> Data Type Conversion2/1
  Delay10/1 -> Data Type Conversion3/1
  Data Type Conversion1/1 -> y1_AXI/1
  Data Type Conversion2/1 -> y2/1
  Data Type Conversion3/1 -> y2_AXI/1

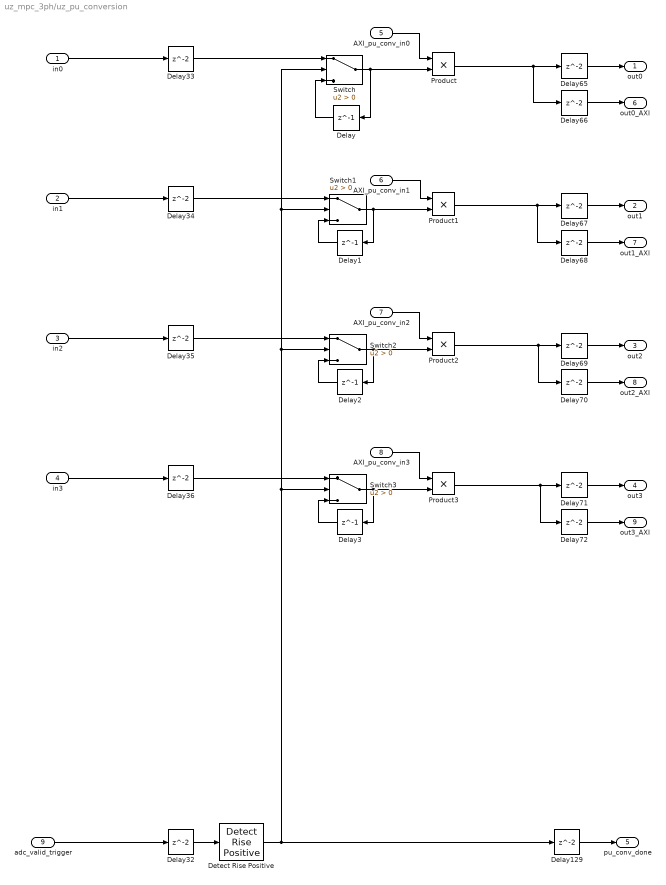
== system uz_mpc_3ph/uz_pu_conversion ==
  in0 : Inport  OutDataTypeStr=fixdt(1,27,15)
  in1 : Inport  Port=2  OutDataTypeStr=fixdt(1,27,15)
  in2 : Inport  Port=3  OutDataTypeStr=fixdt(1,27,15)
  in3 : Inport  Port=4  OutDataTypeStr=fixdt(1,27,15)
  AXI_pu_conv_in0 : Inport  Port=5  OutDataTypeStr=fixdt(0,18,18)
  AXI_pu_conv_in1 : Inport  Port=6  OutDataTypeStr=fixdt(0,18,18)
  AXI_pu_conv_in2 : Inport  Port=7  OutDataTypeStr=fixdt(0,18,18)
  AXI_pu_conv_in3 : Inport  Port=8  OutDataTypeStr=fixdt(0,18,18)
  adc_valid_trigger : Inport  Port=9  OutDataTypeStr=boolean
  Delay{,1..3} (4 alike) : Delay  DelayLength=1
  Delay{32..36,65..72,129} (14 alike) : Delay
  Detect Rise Positive : simulink/Logic and Bit Operations/Detect Rise Positive  vinit=0  OutDataTypeStr=boolean
  Product{,1..3} (4 alike) : Product  OutDataTypeStr=pu_fixdt_type
  Switch{,1..3} (4 alike) : Switch  Criteria=u2 > Threshold
  out0 : Outport
  out1 : Outport  Port=2
  out2 : Outport  Port=3
  out3 : Outport  Port=4
  pu_conv_done : Outport  Port=5  OutDataTypeStr=boolean  LockScale=on
  out0_AXI : Outport  Port=6
  out1_AXI : Outport  Port=7
  out2_AXI : Outport  Port=8
  out3_AXI : Outport  Port=9
  wires:
  AXI_pu_conv_in0/1 -> Product/1
  Product/1 -> Delay65/1, Delay66/1
  AXI_pu_conv_in1/1 -> Product1/1
  Product1/1 -> Delay67/1, Delay68/1
  AXI_pu_conv_in2/1 -> Product2/1
  Product3/1 -> Delay71/1, Delay72/1
  Product2/1 -> Delay69/1, Delay70/1
  AXI_pu_conv_in3/1 -> Product3/1
  Switch/1 -> Product/2, Delay/1
  Delay/1 -> Switch/3
  Switch1/1 -> Product1/2, Delay1/1
  Delay1/1 -> Switch1/3
  Switch2/1 -> Product2/2, Delay2/1
  Delay2/1 -> Switch2/3
  Switch3/1 -> Product3/2, Delay3/1
  Delay3/1 -> Switch3/3
  adc_valid_trigger/1 -> Delay32/1
  Delay32/1 -> Detect Rise Positive/1
  in0/1 -> Delay33/1
  Delay33/1 -> Switch/1
  in1/1 -> Delay34/1
  Delay34/1 -> Switch1/1
  in2/1 -> Delay35/1
  Delay35/1 -> Switch2/1
  in3/1 -> Delay36/1
  Delay36/1 -> Switch3/1
  Delay65/1 -> out0/1
  Delay66/1 -> out0_AXI/1
  Delay67/1 -> out1/1
  Delay68/1 -> out1_AXI/1
  Delay69/1 -> out2/1
  Delay70/1 -> out2_AXI/1
  Delay71/1 -> out3/1
  Delay72/1 -> out3_AXI/1
  Delay129/1 -> pu_conv_done/1
  Detect Rise Positive/1 -> Switch3/2, Switch2/2, Switch1/2, Switch/2, Delay129/1

== system uz_mpc_3ph/uz_sel_currents ==
  ia1_left : Inport
  ia1_right : Inport  Port=2
  ib1_left : Inport  Port=3
  ib1_right : Inport  Port=4
  ic1_left : Inport  Port=5
  ic1_right : Inport  Port=6
  vdc_left : Inport  Port=7
  vdc_right : Inport  Port=8
  right_or_left_AXI : Inport  Port=9
  adc_valid_trigger : Inport  Port=10
  Delay{,1..11,21,28..29} (15 alike) : Delay
  Switch{,1..3} (4 alike) : Switch  Criteria=u2 > Threshold
  ia1 : Outport  VectorParamsAs1DForOutWhenUnconnected=off
  ib1 : Outport  Port=2  VectorParamsAs1DForOutWhenUnconnected=off
  ic1 : Outport  Port=3  VectorParamsAs1DForOutWhenUnconnected=off
  vdc : Outport  Port=4  VectorParamsAs1DForOutWhenUnconnected=off
  selector_ip_done : Outport  Port=5  VectorParamsAs1DForOutWhenUnconnected=off
  wires:
  ia1_left/1 -> Delay/1
  ia1_right/1 -> Delay1/1
  Delay/1 -> Switch/1
  Delay1/1 -> Switch/3
  Switch/1 -> Delay2/1
  Delay2/1 -> ia1/1
  ib1_right/1 -> Delay4/1
  Delay5/1 -> ib1/1
  ib1_left/1 -> Delay3/1
  Delay4/1 -> Switch1/3
  Delay3/1 -> Switch1/1
  Switch1/1 -> Delay5/1
  right_or_left_AXI/1 -> Delay21/1
  Delay28/1 -> Delay29/1
  Delay29/1 -> selector_ip_done/1
  adc_valid_trigger/1 -> Delay28/1
  Delay21/1 -> Switch3/2, Switch2/2, Switch1/2, Switch/2
  Delay8/1 -> ic1/1
  ic1_left/1 -> Delay6/1
  Delay6/1 -> Switch2/1
  ic1_right/1 -> Delay7/1
  Delay7/1 -> Switch2/3
  Switch2/1 -> Delay8/1
  Delay11/1 -> vdc/1
  vdc_left/1 -> Delay9/1
  Delay9/1 -> Switch3/1
  vdc_right/1 -> Delay10/1
  Delay10/1 -> Switch3/3
  Switch3/1 -> Delay11/1

== system uz_mpc_3ph/uz_sel_resolver ==
  omega_m_left : Inport
  omega_m_right : Inport  Port=2
  theta_el_left : Inport  Port=3
  theta_el_right : Inport  Port=4
  right_or_left_AXI : Inport  Port=5
  adc_valid_trigger : Inport  Port=6
  Delay{,1..5,21,28..29} (9 alike) : Delay
  Switch : Switch  Criteria=u2 > Threshold
  Switch1 : Switch  Criteria=u2 > Threshold
  omega_m : Outport  VectorParamsAs1DForOutWhenUnconnected=off
  theta_el : Outport  Port=2  VectorParamsAs1DForOutWhenUnconnected=off
  selector_ip_done : Outport  Port=3  VectorParamsAs1DForOutWhenUnconnected=off
  wires:
  omega_m_left/1 -> Delay/1
  omega_m_right/1 -> Delay1/1
  Delay/1 -> Switch/1
  Delay1/1 -> Switch/3
  Switch/1 -> Delay2/1
  Delay2/1 -> omega_m/1
  theta_el_right/1 -> Delay4/1
  Delay5/1 -> theta_el/1
  theta_el_left/1 -> Delay3/1
  Delay4/1 -> Switch1/3
  Delay3/1 -> Switch1/1
  Switch1/1 -> Delay5/1
  right_or_left_AXI/1 -> Delay21/1
  Delay28/1 -> Delay29/1
  Delay29/1 -> selector_ip_done/1
  adc_valid_trigger/1 -> Delay28/1
  Delay21/1 -> Switch1/2, Switch/2

== system uz_mpc_3ph/ctrl_state_machine/Subsystem ==
  Set : Inport
  Reset : Inport  Port=2
  Constant1 : Constant  Value=0  OutDataTypeStr=uint32  SampleTime=-1
  Data Type Conversion1 : DataTypeConversion  OutDataTypeStr=boolean
  Data Type Conversion2 : DataTypeConversion  OutDataTypeStr=boolean
  Logical Operator : Logic  Operator=NOT  AllPortsSameDT=off  OutDataTypeStr=boolean
  Logical Operator1 : Logic  AllPortsSameDT=off  OutDataTypeStr=boolean
  Logical Operator2 : Logic  Operator=OR  AllPortsSameDT=off  OutDataTypeStr=boolean
  Logical Operator3 : Logic  Operator=NOT  AllPortsSameDT=off  OutDataTypeStr=boolean
  Logical Operator4 : Logic  Operator=OR  AllPortsSameDT=off  OutDataTypeStr=boolean
  Logical Operator5 : Logic  AllPortsSameDT=off  OutDataTypeStr=boolean
  Switch1 : Switch  Criteria=u2 > Threshold  Threshold=1
  Unit Delay : UnitDelay  InitialCondition=1  SampleTime=t_clock  HasFrameUpgradeWarning=on
  Q : Outport  VectorParamsAs1DForOutWhenUnconnected=off
  !Q : Outport  Port=2  VectorParamsAs1DForOutWhenUnconnected=off
  wires:
  Logical Operator/1 -> Logical Operator1/2, Logical Operator5/1
  Reset/1 -> Data Type Conversion2/1
  Constant1/1 -> Switch1/2
  Logical Operator4/1 -> Switch1/1
  Data Type Conversion1/1 -> Logical Operator2/1, Logical Operator4/1
  Switch1/1 -> Q/1, Unit Delay/1, Logical Operator3/1
  Logical Operator3/1 -> !Q/1
  Set/1 -> Data Type Conversion1/1
  Logical Operator2/1 -> Logical Operator1/1
  Unit Delay/1 -> Logical Operator2/2, Logical Operator5/2
  Logical Operator5/1 -> Logical Operator4/2
  Logical Operator1/1 -> Switch1/3
  Data Type Conversion2/1 -> Logical Operator/1

== system uz_mpc_3ph/ctrl_state_machine/Subsystem2 ==
  Set : Inport
  Reset : Inport  Port=2
  Constant1 : Constant  Value=0  OutDataTypeStr=uint32  SampleTime=-1
  Data Type Conversion1 : DataTypeConversion  OutDataTypeStr=boolean
  Data Type Conversion2 : DataTypeConversion  OutDataTypeStr=boolean
  Logical Operator : Logic  Operator=NOT  AllPortsSameDT=off  OutDataTypeStr=boolean
  Logical Operator1 : Logic  AllPortsSameDT=off  OutDataTypeStr=boolean
  Logical Operator2 : Logic  Operator=OR  AllPortsSameDT=off  OutDataTypeStr=boolean
  Logical Operator3 : Logic  Operator=NOT  AllPortsSameDT=off  OutDataTypeStr=boolean
  Logical Operator4 : Logic  Operator=OR  AllPortsSameDT=off  OutDataTypeStr=boolean
  Logical Operator5 : Logic  AllPortsSameDT=off  OutDataTypeStr=boolean
  Switch1 : Switch  Criteria=u2 > Threshold  Threshold=1
  Unit Delay : UnitDelay  SampleTime=t_clock  HasFrameUpgradeWarning=on
  Q : Outport  VectorParamsAs1DForOutWhenUnconnected=off
  !Q : Outport  Port=2  VectorParamsAs1DForOutWhenUnconnected=off
  wires:
  Logical Operator/1 -> Logical Operator1/2, Logical Operator5/1
  Reset/1 -> Data Type Conversion2/1
  Constant1/1 -> Switch1/2
  Logical Operator4/1 -> Switch1/1
  Data Type Conversion1/1 -> Logical Operator2/1, Logical Operator4/1
  Switch1/1 -> Q/1, Unit Delay/1, Logical Operator3/1
  Logical Operator3/1 -> !Q/1
  Set/1 -> Data Type Conversion1/1
  Logical Operator2/1 -> Logical Operator1/1
  Unit Delay/1 -> Logical Operator2/2, Logical Operator5/2
  Logical Operator5/1 -> Logical Operator4/2
  Logical Operator1/1 -> Switch1/3
  Data Type Conversion2/1 -> Logical Operator/1

== system uz_mpc_3ph/ctrl_state_machine/Subsystem4 ==
  Set : Inport
  Reset : Inport  Port=2
  Constant1 : Constant  Value=0  OutDataTypeStr=uint32  SampleTime=-1
  Data Type Conversion1 : DataTypeConversion  OutDataTypeStr=boolean
  Data Type Conversion2 : DataTypeConversion  OutDataTypeStr=boolean
  Logical Operator : Logic  Operator=NOT  AllPortsSameDT=off  OutDataTypeStr=boolean
  Logical Operator1 : Logic  AllPortsSameDT=off  OutDataTypeStr=boolean
  Logical Operator2 : Logic  Operator=OR  AllPortsSameDT=off  OutDataTypeStr=boolean
  Logical Operator3 : Logic  Operator=NOT  AllPortsSameDT=off  OutDataTypeStr=boolean
  Logical Operator4 : Logic  Operator=OR  AllPortsSameDT=off  OutDataTypeStr=boolean
  Logical Operator5 : Logic  AllPortsSameDT=off  OutDataTypeStr=boolean
  Switch1 : Switch  Criteria=u2 > Threshold  Threshold=1
  Unit Delay : UnitDelay  SampleTime=t_clock  HasFrameUpgradeWarning=on
  Q : Outport  VectorParamsAs1DForOutWhenUnconnected=off
  !Q : Outport  Port=2  VectorParamsAs1DForOutWhenUnconnected=off
  wires:
  Logical Operator/1 -> Logical Operator1/2, Logical Operator5/1
  Reset/1 -> Data Type Conversion2/1
  Constant1/1 -> Switch1/2
  Logical Operator4/1 -> Switch1/1
  Data Type Conversion1/1 -> Logical Operator2/1, Logical Operator4/1
  Switch1/1 -> Q/1, Unit Delay/1, Logical Operator3/1
  Logical Operator3/1 -> !Q/1
  Set/1 -> Data Type Conversion1/1
  Logical Operator2/1 -> Logical Operator1/1
  Unit Delay/1 -> Logical Operator2/2, Logical Operator5/2
  Logical Operator5/1 -> Logical Operator4/2
  Logical Operator1/1 -> Switch1/3
  Data Type Conversion2/1 -> Logical Operator/1

== system uz_mpc_3ph/ctrl_state_machine/Subsystem7 ==
  Set : Inport
  Reset : Inport  Port=2
  Constant1 : Constant  Value=0  OutDataTypeStr=uint32  SampleTime=-1
  Data Type Conversion1 : DataTypeConversion  OutDataTypeStr=boolean
  Data Type Conversion2 : DataTypeConversion  OutDataTypeStr=boolean
  Logical Operator : Logic  Operator=NOT  AllPortsSameDT=off  OutDataTypeStr=boolean
  Logical Operator1 : Logic  AllPortsSameDT=off  OutDataTypeStr=boolean
  Logical Operator2 : Logic  Operator=OR  AllPortsSameDT=off  OutDataTypeStr=boolean
  Logical Operator3 : Logic  Operator=NOT  AllPortsSameDT=off  OutDataTypeStr=boolean
  Logical Operator4 : Logic  Operator=OR  AllPortsSameDT=off  OutDataTypeStr=boolean
  Logical Operator5 : Logic  AllPortsSameDT=off  OutDataTypeStr=boolean
  Switch1 : Switch  Criteria=u2 > Threshold  Threshold=1
  Unit Delay : UnitDelay  InitialCondition=1  SampleTime=t_clock  HasFrameUpgradeWarning=on
  Q : Outport  VectorParamsAs1DForOutWhenUnconnected=off
  !Q : Outport  Port=2  VectorParamsAs1DForOutWhenUnconnected=off
  wires:
  Logical Operator/1 -> Logical Operator1/2, Logical Operator5/1
  Reset/1 -> Data Type Conversion2/1
  Constant1/1 -> Switch1/2
  Logical Operator4/1 -> Switch1/1
  Data Type Conversion1/1 -> Logical Operator2/1, Logical Operator4/1
  Switch1/1 -> Q/1, Unit Delay/1, Logical Operator3/1
  Logical Operator3/1 -> !Q/1
  Set/1 -> Data Type Conversion1/1
  Logical Operator2/1 -> Logical Operator1/1
  Unit Delay/1 -> Logical Operator2/2, Logical Operator5/2
  Logical Operator5/1 -> Logical Operator4/2
  Logical Operator1/1 -> Switch1/3
  Data Type Conversion2/1 -> Logical Operator/1

== system uz_mpc_3ph/ctrl_state_machine/limited_counter ==
  limit : Inport
  enb : Inport  Port=2
  Add : Sum  Inputs=-++  AccumDataTypeStr=uint8
  Constant3 : Constant  Value=0  OutDataTypeStr=uint8  SampleTime=-1
  Constant5 : Constant  OutDataTypeStr=uint8  SampleTime=-1
  Constant6 : Constant  Value=0  OutDataTypeStr=uint8  SampleTime=-1
  Delay4 : Delay  DelayLength=1
  Relational Operator1 : RelationalOperator  OutDataTypeStr=boolean  RndMeth=Simplest
  Switch7 : Switch  Criteria=u2 > Threshold
  Switch8 : Switch  Criteria=u2 > Threshold
  cnt : Outport
  wires:
  Constant6/1 -> Switch8/3
  Constant3/1 -> Switch7/3
  Switch8/1 -> Add/1  "trigger"
  Delay4/1 -> Add/3, Relational Operator1/1, Switch8/1
  Switch7/1 -> Add/2  "trigger"
  Constant5/1 -> Switch7/1
  Relational Operator1/1 -> Switch8/2
  Add/1 -> cnt/1, Delay4/1
  limit/1 -> Relational Operator1/2
  enb/1 -> Switch7/2

== system uz_mpc_3ph/ctrl_state_machine/resetable_counter ==
  enb : Inport
  rst : Inport  Port=2
  Add : Sum  Inputs=-++  AccumDataTypeStr=uint8
  Add1 : Sum  Inputs=+-  AccumDataTypeStr=uint8
  Constant1 : Constant  Value=0  OutDataTypeStr=uint8  SampleTime=-1
  Constant3 : Constant  Value=0  OutDataTypeStr=uint8  SampleTime=-1
  Constant5 : Constant  OutDataTypeStr=uint8  SampleTime=-1
  Constant6 : Constant  Value=0  OutDataTypeStr=uint8  SampleTime=-1
  Delay4 : Delay  DelayLength=1
  Switch7 : Switch  Criteria=u2 > Threshold
  Switch8 : Switch  Criteria=u2 > Threshold
  cnt : Outport
  wires:
  Constant6/1 -> Switch8/3
  Constant3/1 -> Switch7/3
  Switch8/1 -> Add/1  "trigger"
  Switch7/1 -> Add/2  "trigger"
  Constant5/1 -> Switch7/1
  Add/1 -> cnt/1, Delay4/1
  enb/1 -> Switch7/2
  Constant1/1 -> Add1/2
  Add1/1 -> Switch8/1
  Delay4/1 -> Add/3, Add1/1
  rst/1 -> Switch8/2
